simulink model "ADXL345_IMU"  (R2017a)
settings: Solver=FixedStepDiscrete  StartTime=0.0  StopTime=0.01  RelTol=1e-3
PostLoadFcn:
  | ChipSelect = 1;  % choose I2C comms
  | AddressAlt  = 1;  % use default address
  | 
  | if AddressAlt == 1
  | SlvAddr = uint8(hex2dec('1D'));  % ADDR ALT = 1
  | else
  | SlvAddr = uint8(hex2dec('53'));  % ADDR ALT = 0
  | end
  | 
  | AccelXRegAddr = uint8(hex2dec('32'));
  | AccelYRegAddr = uint8(hex2dec('34'));
  | AccelZRegAddr = uint8(hex2dec('36'));
  | 
  | fifoCfgRegAddr = uint8(hex2dec('38'));
  | fifoCfgRegData = uint8(bin2dec('00000100'));
  | 
  | fifoStatusReg = uint8(hex2dec('39'));
  | 
  | deviceAddr = fi(SlvAddr,0,7,0);
settings Model: DataTypeOverride=Off  Creator=skuznick  LastModifiedBy=skuznick
settings DataIOCC: SaveOutput=off  SaveTime=off
settings OptimizationCC: BlockReduction=off  ConditionallyExecuteInputs=off  DefaultParameterBehavior=Inlined
settings DebuggingCC: AlgebraicLoopMsg=error  SingleTaskRateTransMsg=error
settings HardwareCC: ProdBitPerPointer=32  ProdBitPerSizeT=32  ProdBitPerPtrDiffT=32  ProdLargestAtomicFloat=None  ProdIntDivRoundTo=Undefined  ProdEndianess=Unspecified  ProdWordSize=32  ProdHWDeviceType=ASIC/FPGA->ASIC/FPGA  ProdEqTarget=off

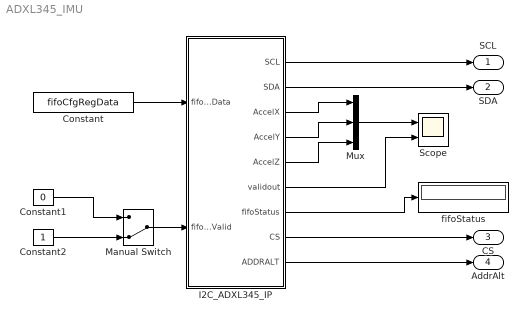
== system ADXL345_IMU ==
  Constant : Constant  Value=fifoCfgRegData  OutDataTypeStr=uint8  SampleTime=1/400e3
  Constant1 : Constant  Value=0  OutDataTypeStr=boolean  SampleTime=-1
  Constant2 : Constant  OutDataTypeStr=boolean  SampleTime=-1
  I2C_ADXL345_IP : Subsystem  TreatAsAtomicUnit=on
  Manual Switch : ManualSwitch  CurrentSetting=0
  Mux : Mux  Inputs=3
  Scope : Scope  NumInputPorts=2
  fifoStatus : Display
  SCL : Outport
  SDA : Outport  Port=2
  CS : Outport  Port=3
  AddrAlt : Outport  Port=4
  wires:
  I2C_ADXL345_IP/2(SDA) -> SDA/1
  I2C_ADXL345_IP/1(SCL) -> SCL/1
  I2C_ADXL345_IP/8(CS) -> CS/1
  I2C_ADXL345_IP/9(ADDRALT) -> AddrAlt/1
  Manual Switch/1 -> I2C_ADXL345_IP/2(fifoCfgValid)
  Constant1/1 -> Manual Switch/1
  Constant2/1 -> Manual Switch/2
  Constant/1 -> I2C_ADXL345_IP/1(fifoCfgData)
  I2C_ADXL345_IP/6(validout) -> Scope/2
  Mux/1 -> Scope/1
  I2C_ADXL345_IP/4(AccelY) -> Mux/2
  I2C_ADXL345_IP/3(AccelX) -> Mux/1
  I2C_ADXL345_IP/5(AccelZ) -> Mux/3
  I2C_ADXL345_IP/7(fifoStatus) -> fifoStatus/1

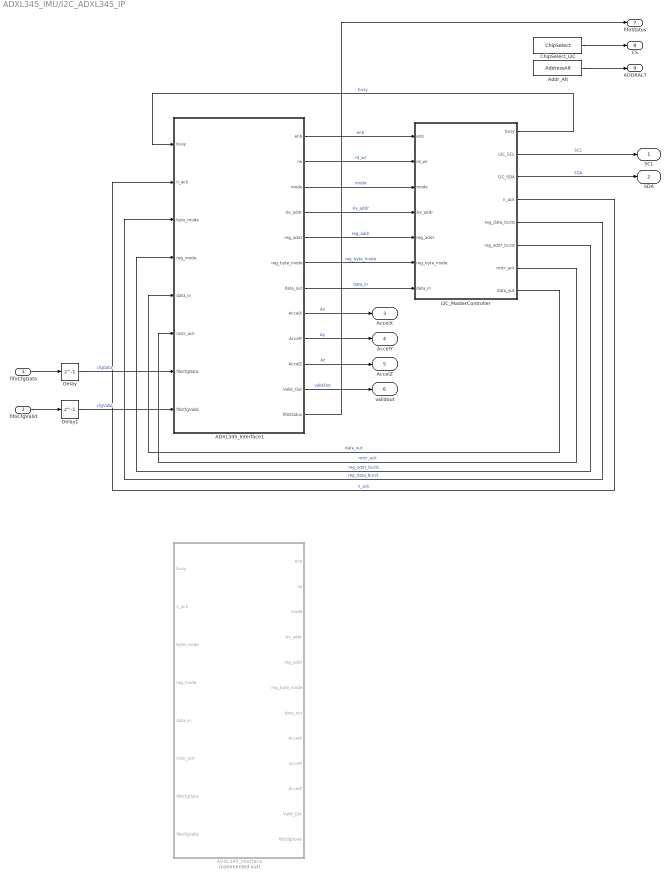
== system ADXL345_IMU/I2C_ADXL345_IP ==
  fifoCfgData : Inport
  fifoCfgValid : Inport  Port=2
  ADXL345_Interface : Stateflow chart  Commented=on  TreatAsAtomicUnit=on
  ADXL345_Interface1 : Stateflow chart  TreatAsAtomicUnit=on
  Addr_Alt : Constant  Value=AddressAlt  OutDataTypeStr=boolean  SampleTime=-1
  ChipSelect_I2C : Constant  Value=ChipSelect  OutDataTypeStr=boolean  SampleTime=-1
  Delay : Delay  DelayLength=1  InitialCondition=0
  Delay1 : Delay  DelayLength=1  InitialCondition=0
  I2C_MasterController : Subsystem
  SCL : Outport
  SDA : Outport  Port=2
  AccelX : Outport  Port=3
  AccelY : Outport  Port=4
  AccelZ : Outport  Port=5
  validout : Outport  Port=6
  fifoStatus : Outport  Port=7
  CS : Outport  Port=8
  ADDRALT : Outport  Port=9
  wires:
  ADXL345_Interface1/7(data_out) -> I2C_MasterController/7(data_in)  "data_in"
  I2C_MasterController/8(data_out) -> ADXL345_Interface1/5(data_in)  "data_out"
  I2C_MasterController/7(mstr_ack) -> ADXL345_Interface1/6(mstr_ack)  "mstr_ack"
  I2C_MasterController/4(n_ack) -> ADXL345_Interface1/2(n_ack)  "n_ack"
  I2C_MasterController/5(reg_data_burst) -> ADXL345_Interface1/3(byte_mode)  "reg_data_burst"
  I2C_MasterController/6(reg_addr_burst) -> ADXL345_Interface1/4(reg_mode)  "reg_addr_burst"
  I2C_MasterController/1(busy) -> ADXL345_Interface1/1(busy)  "busy"
  I2C_MasterController/3(I2C_SDA) -> SDA/1  "SDA"
  I2C_MasterController/2(I2C_SCL) -> SCL/1  "SCL"
  ADXL345_Interface1/6(reg_byte_mode) -> I2C_MasterController/6(reg_byte_mode)  "reg_byte_mode"
  ADXL345_Interface1/5(reg_addr) -> I2C_MasterController/5(reg_addr)  "reg_addr"
  ADXL345_Interface1/4(slv_addr) -> I2C_MasterController/4(slv_addr)  "slv_addr"
  ADXL345_Interface1/3(mode) -> I2C_MasterController/3(mode)  "mode"
  ADXL345_Interface1/2(rw) -> I2C_MasterController/2(rd_wr)  "rd_wr"
  ADXL345_Interface1/1(enb) -> I2C_MasterController/1(enb)  "enb"
  Delay/1 -> ADXL345_Interface1/7(fifoCfgData)  "cfgData"
  Delay1/1 -> ADXL345_Interface1/8(fifoCfgValid)  "cfgValid"
  fifoCfgData/1 -> Delay/1
  fifoCfgValid/1 -> Delay1/1
  ChipSelect_I2C/1 -> CS/1
  Addr_Alt/1 -> ADDRALT/1
  ADXL345_Interface1/9(AccelY) -> AccelY/1  "Ay"
  ADXL345_Interface1/10(AccelZ) -> AccelZ/1  "Az"
  ADXL345_Interface1/11(Valid_Out) -> validout/1  "validOut"
  ADXL345_Interface1/8(AccelX) -> AccelX/1  "Ax"
  ADXL345_Interface1/12(fifoStatus) -> fifoStatus/1

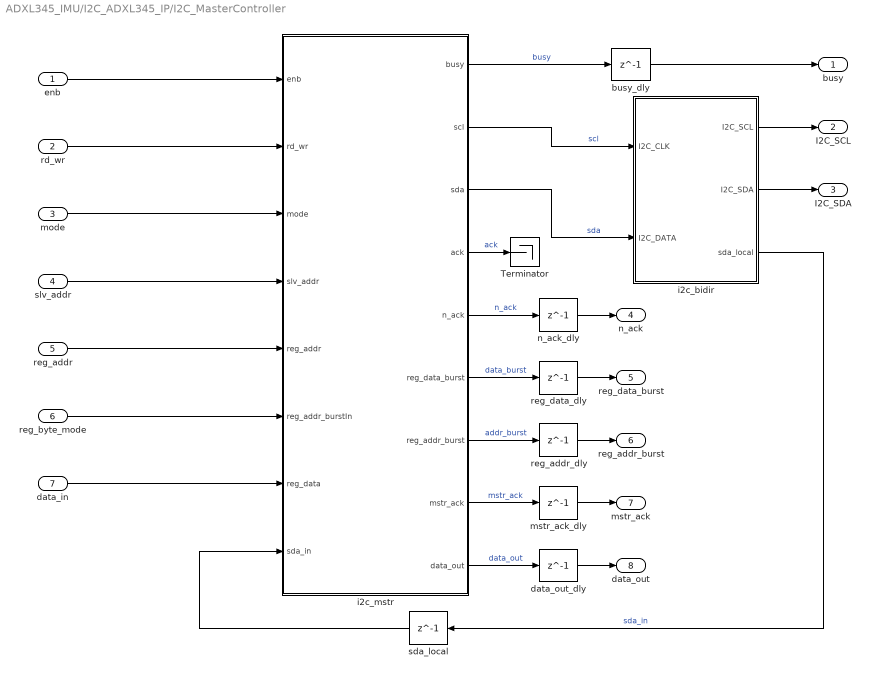
== system ADXL345_IMU/I2C_ADXL345_IP/I2C_MasterController ==
  enb : Inport
  rd_wr : Inport  Port=2
  mode : Inport  Port=3
  slv_addr : Inport  Port=4
  reg_addr : Inport  Port=5
  reg_byte_mode : Inport  Port=6
  data_in : Inport  Port=7
  Terminator : Terminator
  busy_dly : Delay  DelayLength=1
  data_out_dly : Delay  DelayLength=1
  i2c_bidir : Subsystem  TreatAsAtomicUnit=on
  i2c_mstr : Stateflow chart  TreatAsAtomicUnit=on
  mstr_ack_dly : Delay  DelayLength=1
  n_ack_dly : Delay  DelayLength=1
  reg_addr_dly : Delay  DelayLength=1
  reg_data_dly : Delay  DelayLength=1
  sda_local : Delay  DelayLength=1
  busy : Outport
  I2C_SCL : Outport  Port=2
  I2C_SDA : Outport  Port=3
  n_ack : Outport  Port=4
  reg_data_burst : Outport  Port=5
  reg_addr_burst : Outport  Port=6
  mstr_ack : Outport  Port=7
  data_out : Outport  Port=8
  wires:
  data_out_dly/1 -> data_out/1
  mstr_ack_dly/1 -> mstr_ack/1
  i2c_mstr/9(data_out) -> data_out_dly/1  "data_out"
  i2c_mstr/8(mstr_ack) -> mstr_ack_dly/1  "mstr_ack"
  busy_dly/1 -> busy/1
  n_ack_dly/1 -> n_ack/1
  reg_data_dly/1 -> reg_data_burst/1
  reg_addr_dly/1 -> reg_addr_burst/1
  i2c_mstr/1(busy) -> busy_dly/1  "busy"
  rd_wr/1 -> i2c_mstr/2(rd_wr)
  mode/1 -> i2c_mstr/3(mode)
  data_in/1 -> i2c_mstr/7(reg_data)
  enb/1 -> i2c_mstr/1(enb)
  slv_addr/1 -> i2c_mstr/4(slv_addr)
  reg_byte_mode/1 -> i2c_mstr/6(reg_addr_burstIn)
  reg_addr/1 -> i2c_mstr/5(reg_addr)
  i2c_bidir/1(I2C_SCL) -> I2C_SCL/1
  i2c_bidir/2(I2C_SDA) -> I2C_SDA/1
  i2c_mstr/4(ack) -> Terminator/1  "ack"
  i2c_mstr/2(scl) -> i2c_bidir/1(I2C_CLK)  "scl"
  i2c_bidir/3(sda_local) -> sda_local/1  "sda_in"
  sda_local/1 -> i2c_mstr/8(sda_in)
  i2c_mstr/3(sda) -> i2c_bidir/2(I2C_DATA)  "sda"
  i2c_mstr/5(n_ack) -> n_ack_dly/1  "n_ack"
  i2c_mstr/6(reg_data_burst) -> reg_data_dly/1  "data_burst"
  i2c_mstr/7(reg_addr_burst) -> reg_addr_dly/1  "addr_burst"

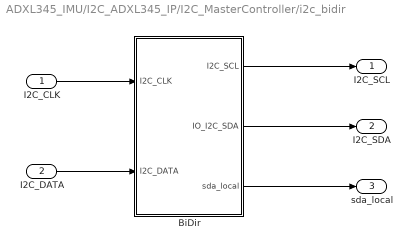
== system ADXL345_IMU/I2C_ADXL345_IP/I2C_MasterController/i2c_bidir ==
  I2C_CLK : Inport
  I2C_DATA : Inport  Port=2
  BiDir : Subsystem  TreatAsAtomicUnit=on
  I2C_SCL : Outport
  I2C_SDA : Outport  Port=2
  sda_local : Outport  Port=3
  wires:
  BiDir/2(IO_I2C_SDA) -> I2C_SDA/1
  I2C_CLK/1 -> BiDir/1(I2C_CLK)
  I2C_DATA/1 -> BiDir/2(I2C_DATA)
  BiDir/1("I2C_SCL ") -> I2C_SCL/1
  BiDir/3(sda_local) -> sda_local/1

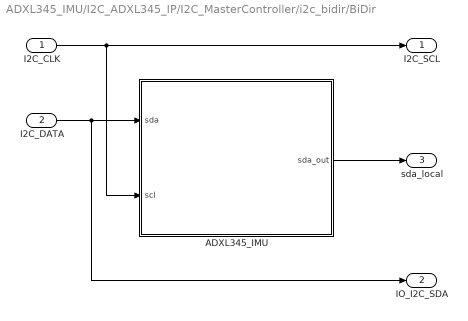
== system ADXL345_IMU/I2C_ADXL345_IP/I2C_MasterController/i2c_bidir/BiDir ==
  I2C_CLK : Inport  OutDataTypeStr=boolean
  I2C_DATA : Inport  Port=2  OutDataTypeStr=boolean
  ADXL345_IMU : Stateflow chart  TreatAsAtomicUnit=on
  "I2C_SCL " : Outport  OutDataTypeStr=boolean
  IO_I2C_SDA : Outport  Port=2  OutDataTypeStr=boolean
  sda_local : Outport  Port=3  OutDataTypeStr=boolean
  wires:
  ADXL345_IMU/1(sda_out) -> sda_local/1
  I2C_CLK/1 -> "I2C_SCL "/1, ADXL345_IMU/2(scl)
  I2C_DATA/1 -> IO_I2C_SDA/1, ADXL345_IMU/1(sda)

== stateflow chart ADXL345_IMU/I2C_ADXL345_IP/ADXL345_Interface1 ==
  settings: executeAtInitialization=1
  state init
    %initstate
    Valid_Out = false;
  note: I2C Configuration for ADXL345
  state idle
    %idlestate
    enb 	= 0;
    rw 		= 0;
    mode 	= 0;
    inc_in  = 0;
    wait 	= 0;
    cnt = 0;
    reg_byte_mode = 0;
  note: 0x32 50 DATAX0 R 00000000 X-Axis Data 0
      | 0x33 51 DATAX1 R 00000000 X-Axis Data 1
      | 0x34 52 DATAY0 R 00000000 Y-Axis Data 0
      | 0x35 53 DATAY1 R 00000000 Y-Axis Data 1
      | 0x36 54 DATAZ0 R 00000000 Z-Axis Data 0
      | 0x37 55 DATAZ1 R 00000000 Z-Axis Data 1
  state set_config [commented out]
    enb = 1;
    rw = 0;
    mode = 0;
    reg_byte_mode = 0;
    slv_addr = SlvAddr;
    reg_addr = fifoCfgRegAddr;
    data_out = fifoCfgData;
  state waitforNotBusy [commented out]
  state getFifoStatus [commented out]
    entry:
    enb = 1;
    rw = 1;
    mode = 0;
    slv_addr = SlvAddr;
    reg_addr =  fifoStatusReg;
  state read_fifoReg [commented out]
    fifoStatus = uint8(data_in);
  note: fifoStatus is an example of
      | doing a 1-byte READ
  state check_cfg
    en: enb = 0;
  state read_accelX_registers0
    entry:
    enb = 1;
    rw = 1;
    mode = 1;
    slv_addr = SlvAddr;
    reg_byte_mode = 0;
    reg_addr =  AccelXRegAddr;
    Valid_Out = false;
  state accelX_LSB
    enb = 1;
    tempVal = uint16(data_in);
  state toggle
    mode = 0;
  state accelX_MSB
    enb = 0;
    AccelX = tempVal + uint16(data_in << 8);
  state read_accelY_registers0
    enb = 1;
    rw = 1;
    mode = 1;
    slv_addr = SlvAddr;
    reg_byte_mode = 0;
    reg_addr =  AccelYRegAddr;
  state accelY_LSB
    enb = 1;
    tempVal = uint16(data_in);
  state toggle1
    mode = 0;
  state accelY_MSB
    enb = 0;
    AccelY = tempVal + uint16(data_in << 8);
  state read_accelZ_registers0
    enb = 1;
    rw = 1;
    mode = 1;
    slv_addr = SlvAddr;
    reg_byte_mode = 0;
    reg_addr =  AccelZRegAddr;
  state accelZ_LSB
    enb = 1;
    tempVal = uint16(data_in);
  state toggle2
    mode = 0;
  state accelZ_MSB
    enb = 0;
    AccelZ = tempVal + uint16(data_in << 8);
  state Valid
    en: enb = 0;
    cnt = 0;
    Valid_Out = 1;
    du: cnt = cnt + 1;
  (default) -> init
  init -> idle
  check_cfg -> idle
  accelX_LSB -> idle [order 1] : [n_ack==1]
  idle -> set_config [commented out] : [busy==0 & fifoCfgValid == 1]
  idle -> read_accelX_registers0
  set_config -> waitforNotBusy [commented out] : [busy==1]
  waitforNotBusy -> getFifoStatus [commented out] : [busy==0]
  getFifoStatus -> read_fifoReg [commented out] : [mstr_ack==1]
  read_fifoReg -> read_accelX_registers0 [commented out] : [busy==0]
  read_accelX_registers0 -> check_cfg [order 2] : [n_ack == 1]
  accelX_MSB -> check_cfg [order 2] : [n_ack==1]
  accelZ_MSB -> check_cfg [order 1] : [n_ack==1]
  Valid -> check_cfg : [cnt >= 1000]
  accelY_MSB -> check_cfg [order 2] : [n_ack==1]
  read_accelX_registers0 -> accelX_LSB [order 1] : [mstr_ack==1]
  accelX_LSB -> toggle [order 2] : [mstr_ack==0]
  toggle -> accelX_MSB : [mstr_ack==1]
  accelX_MSB -> read_accelY_registers0 [order 1] : [busy==0]
  read_accelY_registers0 -> accelY_LSB : [mstr_ack==1]
  accelY_LSB -> toggle1 : [mstr_ack==0]
  toggle1 -> accelY_MSB : [mstr_ack==1]
  accelY_MSB -> read_accelZ_registers0 [order 1] : [busy==0 & n_ack==0]
  read_accelZ_registers0 -> accelZ_LSB : [mstr_ack==1]
  accelZ_LSB -> toggle2 : [mstr_ack==0]
  toggle2 -> accelZ_MSB : [mstr_ack==1]
  accelZ_MSB -> Valid [order 2]
  data: enb output boolean size=1; rw output boolean size=1; mode output boolean size=1; slv_addr output uint8; reg_addr output uint8; reg_byte_mode output boolean size=1; data_out output uint8; busy input; inc_in local uint8; n_ack input; byte_mode input boolean size=1; reg_mode input boolean size=1; cnt local uint32; wait local uint16; data_in input uint8 size=1; mstr_ack input; AccelX output uint16; AccelY output uint16; AccelZ output uint16; SlvAddr parameter uint8; AccelXRegAddr parameter uint8; AccelYRegAddr parameter uint8; AccelZRegAddr parameter uint8; Valid_Out output boolean; fifoCfgRegAddr parameter uint8; fifoCfgData input uint8; fifoCfgValid input boolean; tempVal local uint16; fifoStatus output uint8; fifoStatusReg parameter uint8

== stateflow chart ADXL345_IMU/I2C_ADXL345_IP/I2C_MasterController/i2c_mstr ==
  settings: executeAtInitialization=1
  note: I2C Master Controller
  state idle
    entry:
    scl(:) = 1;
    sda(:) = 1;
    busy(:)  = 0;
  state stop_ext
    entry:
    scl (:) = 1;
    sda(:) = 1;
    ack(:) = 0;
  state ready
    entry:
    scl(:) = 1;
    sda(:) = 1;
    data_out(:) = 0;
  state stop
    entry:
    sda(:) = 0;
  state start_n
    entry:
    scl(:) = 1;
    sda(:) = 0;
    bit_cnt(:) = 7;
    busy(:) = 1;
    reg_byte_cnt =1;
  state scl_ext_p
    entry:
    scl(:) = 1;
    sda(:) = 0;
    ack(:) = 0;
  state start_p
    entry:
    sda(:) = 0;
  state scl_ext_n
    entry:
    scl(:) = 0;
    sda(:) = 0;
    ack(:) = 0;
    mstr_ack(:) = 0;
  state Increment_Byte_count1
    entry:
    scl(:) = 1;
    bit_cnt = 8;
    mstr_ack(:) =0;
    reg_data_burst(:) = 1;
    data_out(:) = 0;
  state mastr_ack_data_cnf
    entry:
    scl(:) = 1;
    sda(:) = 0;
    mstr_ack (:) = 1;
  state cmd_slave_addr_n
    entry:
    scl(:) = 0;
    sda(:) = bitget(slv_addr(:),bit_cnt);
  state ack_data_cnf
    entry:
    scl(:) = 1;
    ack (:) = 1;
  state cmd_slave_addr_p
    entry:
    scl(:) = 1;
    bit_cnt = bit_cnt-1;
  state Increment_Byte_count
    entry:
    scl(:) = 1;
    bit_cnt = 8;
    ack (:) = 1;
    reg_data_burst(:) = 1;
  state mastr_ack_data
    entry:
    scl(:) = 0;
    sda(:) = 0;
    mstr_ack(:) = 1;
  state write_n
    entry:
    scl(:) = 0;
    sda(:) = 0;
  state ack_data
    entry:
    scl(:) = 0;
    sda(:) = 1;
    ack(:) = 1;
  state cmd_reg_read_data_p
    entry:
    scl(:) = 1;
    bit_cnt = bit_cnt-1;
  state write_p
    entry:
    scl(:) = 1;
    sda(:) = 0;
  state cmd_reg_data_p
    entry:
    scl(:) = 1;
    bit_cnt = bit_cnt-1;
  state ack_slv
    entry:
    scl(:) = 0;
    ack(:) = 1;
    sda(:) = 1;
  state error_ack
    entry:
    scl(:) = 0;
    sda(:) = 1;
    n_ack(:) = 1;
  state cmd_reg_read_data_n
    entry:
    scl(:) = 0;
    if sda_in == 1;
    data_out = bitset(data_out,bit_cnt);
    end
    %data_out(bit_cnt) = sda_in;
    %mstr_ack(:) = 0
    ack(:) = 0;
  state ack_slv_cnf
    entry:
    scl(:)= 1;
    ack(:) = 1;
    bit_cnt = 8;
  state cmd_reg_data_n
    entry:
    scl(:) = 0;
    sda(:) = bitget(reg_data,bit_cnt);
    ack(:) = 0;
    reg_data_burst(:) = 0;
  state ack_addr_m_cnf
    entry:
    scl(:) = 1;
    bit_cnt = 8;
    ack(:) = 1;
  state cmd_reg_addr_n
    entry:
    scl(:) = 0;
    ack(:) = 0;
    sda(:) = bitget(reg_addr,bit_cnt);
    reg_addr_burst(:)=0;
  state delay
    entry:
    scl(:) = 0;
    sda(:) = 1;
  state repeat_strt_n
    entry:
    scl(:) = 1;
    sda(:) = 0;
    bit_cnt(:) = 7;
    busy(:) = 1;
    reg_byte_cnt =1;
  state cmd_reg_addr_p
    entry:
    scl(:)= 1;
    bit_cnt = bit_cnt-1;
  state ready_repeated
    entry:
    scl(:) = 1;
    sda(:) = 1;
  state ack_addr_m
    entry:
    scl(:) = 0;
    ack (:) = 1;
    sda(:) = 1;
  state repeat_strt_p
    entry:
    sda(:) = 0;
  state ready_repeated_dummy
    entry:
    scl(:) = 1;
    sda(:) = 1;
  state ack_addrm1
    entry:
    scl(:) = 1;
    ack(:) = 1;
    bit_cnt = 8;
    reg_addr_burst(:)=1;
  state cmd_slave_addr_n1
    entry:
    scl(:) = 0;
    sda(:) = bitget(slv_addr(:),bit_cnt);
  state cmd_slave_addr_p1
    entry:
    scl(:) = 1;
    bit_cnt = bit_cnt-1;
  state read_n
    entry:
    scl(:) = 0;
    sda(:) = 1;
  state read_p
    entry:
    scl(:) = 1;
    sda(:) = 1;
    bit_cnt = 8;
  state ack_slv1
    entry:
    scl(:) = 0;
    ack(:) = 1;
    sda(:) = 1;
  state ack_slv_cnf1
    entry:
    scl(:)= 1;
    ack(:) = 1;
    bit_cnt = 8;
  (default) -> idle
  stop_ext -> idle
  error_ack -> idle
  idle -> ready : [enb==1]
  stop -> stop_ext
  ready -> start_n
  scl_ext_p -> stop
  start_n -> start_p
  scl_ext_n -> scl_ext_p
  start_p -> cmd_slave_addr_n
  mastr_ack_data_cnf -> scl_ext_n [order 2]
  mastr_ack_data_cnf -> Increment_Byte_count1 [order 1] : [mode ==1]
  cmd_slave_addr_p -> cmd_slave_addr_n [order 1] : [bit_cnt > 0]
  ack_data_cnf -> scl_ext_n
  cmd_slave_addr_n -> cmd_slave_addr_p
  mastr_ack_data -> mastr_ack_data_cnf
  Increment_Byte_count1 -> cmd_reg_read_data_n
  ack_data -> ack_data_cnf [order 2] : [sda_in == 0]
  cmd_slave_addr_p -> write_n [order 2]
  Increment_Byte_count -> cmd_reg_data_n
  cmd_reg_read_data_p -> mastr_ack_data [order 2]
  ack_data -> Increment_Byte_count [order 1] : [mode == 1]
  ack_data -> error_ack [order 3]
  write_n -> write_p
  cmd_reg_read_data_p -> cmd_reg_read_data_n [order 1] : [bit_cnt > 0]
  cmd_reg_data_p -> ack_data [order 2]
  cmd_reg_read_data_n -> cmd_reg_read_data_p
  write_p -> ack_slv
  ack_slv -> error_ack [order 2]
  cmd_reg_data_p -> cmd_reg_data_n [order 1] : [bit_cnt > 0]
  cmd_reg_data_n -> cmd_reg_data_p
  ack_slv -> ack_slv_cnf [order 1] : [sda_in == 0]
  ack_addr_m -> error_ack [order 3]
  ack_slv1 -> error_ack [order 2]
  ack_slv_cnf1 -> cmd_reg_read_data_n
  ack_slv_cnf -> cmd_reg_addr_n
  ack_addr_m -> ack_addr_m_cnf [order 2] : [sda_in == 0]
  ack_addr_m_cnf -> cmd_reg_data_n [order 1] : [rd_wr ==0]
  ack_addrm1 -> cmd_reg_addr_n
  ack_addr_m_cnf -> delay [order 2] : [rd_wr == 1]
  cmd_reg_addr_p -> cmd_reg_addr_n [order 1] : [bit_cnt > 0]
  cmd_reg_addr_n -> cmd_reg_addr_p
  delay -> ready_repeated
  ready_repeated_dummy -> repeat_strt_n
  cmd_reg_addr_p -> ack_addr_m [order 2]
  repeat_strt_n -> repeat_strt_p
  ready_repeated -> ready_repeated_dummy
  ack_addr_m -> ack_addrm1 [order 1] : [reg_addr_burstIn ==1]
  repeat_strt_p -> cmd_slave_addr_n1
  cmd_slave_addr_p1 -> cmd_slave_addr_n1 [order 1] : [bit_cnt > 0]
  cmd_slave_addr_n1 -> cmd_slave_addr_p1
  cmd_slave_addr_p1 -> read_n [order 2]
  read_n -> read_p
  read_p -> ack_slv1
  ack_slv1 -> ack_slv_cnf1 [order 1] : [sda_in == 0]
  data: enb input boolean size=1; rd_wr input boolean size=1; mode input boolean size=1; busy output boolean size=1; bit_cnt local uint8; scl output boolean size=1; sda output boolean size=1; slv_addr input uint8; reg_addr input uint8; reg_addr_burstIn input boolean size=1; reg_data input uint8; sda_in input boolean size=1; ack output boolean size=1; n_ack output boolean size=1; reg_byte_cnt local uint8; reg_data_burst output boolean size=1; reg_addr_burst output boolean size=1; mstr_ack output boolean size=1; data_out output fixdt(0,8,0) size=1

== stateflow chart ADXL345_IMU/I2C_ADXL345_IP/ADXL345_Interface ==
  settings: executeAtInitialization=1
  state init
    %initstate
    enb 	= 0;
    rw 		= 0;
    mode 	= 0;
    inc_in  = 0;
    wait 	= 0;
    cnt = 0;
    Valid_Out = false;
    fifoCfgDone = 0;
  state set_config
    enb = 1;
    rw = 0;
    mode = 0;
    reg_byte_mode = 0;
    slv_addr = SlvAddr;
    reg_addr = fifoCfgRegAddr;
    data_out = fifoCfgData;
  note: I2C Configuration for ADXL345
  note: 0x32 50 DATAX0 R 00000000 X-Axis Data 0
      | 0x33 51 DATAX1 R 00000000 X-Axis Data 1
      | 0x34 52 DATAY0 R 00000000 Y-Axis Data 0
      | 0x35 53 DATAY1 R 00000000 Y-Axis Data 1
      | 0x36 54 DATAZ0 R 00000000 Z-Axis Data 0
      | 0x37 55 DATAZ1 R 00000000 Z-Axis Data 1
  state read_accelX_registers
    fifoCfgDone = 1;
    enb = 1;
    rw = 1;
    mode = 1;
    slv_addr = SlvAddr;
    reg_byte_mode = 0;
    reg_addr =  AccelXRegAddr;
  state check_cfg
    en: enb = 0;
    fifoCfgDone = 0;
  state accelX_HSB
    enb = 0;
    AccelX = AccelX & (data_in << 8);
  state accelX_LSB
    enb=1;
    mode = 0;
    AccelX = uint16(data_in);
  state read_accelY_registers
    enb = 1;
    rw = 1;
    mode = 1;
    slv_addr = SlvAddr;
    reg_byte_mode = 0;
    reg_addr =  AccelYRegAddr;
  state accelY_LSB
    enb = 1;
    mode = 0;
    AccelY = data_in;
  state accelY_HSB
    enb = 0;
    AccelY = AccelY & (data_in << 8);
  state read_accelZ_registers
    enb = 1;
    rw = 1;
    mode = 1;
    slv_addr = SlvAddr;
    reg_byte_mode = 0;
    reg_addr =  AccelZRegAddr;
  state accelZ_LSB
    enb = 1;
    mode = 0;
    AccelZ = uint16(data_in);
  state accelZ_HSB
    enb = 0;
    AccelZ = AccelZ & (data_in << 8);
  state Valid
    en: enb = 0;
    cnt = 0;
    Valid_Out = 1;
    du: cnt = cnt + 1;
  (default) -> init
  init -> set_config : [busy==0]
  read_accelX_registers -> init [order 2] : [n_ack == 1]
  set_config -> init [order 2] : [n_ack == 1]
  set_config -> read_accelX_registers [order 1] : [busy==0 & n_ack == 0]
  check_cfg -> set_config [order 1] : [fifoCfgValid == 1]
  check_cfg -> read_accelX_registers [order 2]
  read_accelX_registers -> accelX_LSB [order 1] : [mstr_ack==1 ]
  accelX_LSB -> read_accelX_registers [order 2] : [n_ack==1]
  Valid -> check_cfg : [cnt >= 500]
  accelX_HSB -> read_accelX_registers [order 1] : [n_ack == 1]
  accelX_LSB -> accelX_HSB [order 1] : [byte_mode == 1& mstr_ack==1]
  accelX_HSB -> read_accelY_registers [order 2] : [busy==0 & n_ack == 0]
  read_accelY_registers -> accelY_LSB : [mstr_ack==1 ]
  accelY_LSB -> read_accelY_registers [order 2] : [n_ack==1]
  accelY_HSB -> read_accelY_registers [order 1] : [n_ack == 1]
  accelY_LSB -> accelY_HSB [order 1] : [byte_mode == 1& mstr_ack==1]
  accelY_HSB -> read_accelZ_registers [order 2] : [busy==0 & n_ack == 0]
  read_accelZ_registers -> accelZ_LSB : [mstr_ack == 1 ]
  accelZ_LSB -> read_accelZ_registers [order 1] : [n_ack==1]
  accelZ_HSB -> read_accelZ_registers [order 1] : [n_ack == 1]
  accelZ_LSB -> accelZ_HSB [order 2] : [byte_mode == 1& mstr_ack==1]
  accelZ_HSB -> Valid [order 2] : [busy==0 & n_ack == 0]
  data: enb output boolean size=1; rw output boolean size=1; mode output boolean size=1; slv_addr output uint8; reg_addr output uint8; reg_byte_mode output boolean size=1; data_out output uint8; busy input; inc_in local uint8; n_ack input; byte_mode input boolean size=1; reg_mode input boolean size=1; cnt local uint32; wait local uint16; data_in input uint8 size=1; mstr_ack input; AccelX output uint16; AccelY output uint16; AccelZ output uint16; SlvAddr parameter uint8; AccelXRegAddr parameter uint8; AccelYRegAddr parameter uint8; AccelZRegAddr parameter uint8; Valid_Out output boolean; fifoCfgRegAddr parameter uint8; fifoCfgRegData parameter uint8; fifoCfgData input uint8; fifoCfgValid input boolean; fifoCfgDone output boolean

== stateflow chart ADXL345_IMU/I2C_ADXL345_IP/I2C_MasterController/i2c_bidir/BiDir/ADXL345_IMU ==
  state init
    entry:
    rd_cnt = 0;
    reg_idx = 0;
  state regdata = sendregdata(reg) [function]
    (default) -> (junction 86)
    (junction 86) -> (junction 89) [order 1] : [reg ==AccelXRegAddr]
    (junction 86) -> (junction 88) [order 2]
    (junction 89) -> (junction 90) : {regdata = hex2dec('D2');}
    (junction 90) -> (junction 99)
    (junction 99) -> (junction 112)
    (junction 88) -> (junction 97) [order 1] : [reg==AccelYRegAddr]
    (junction 97) -> (junction 111) : {regdata = hex2dec('E1');}
    (junction 88) -> (junction 91) [order 2]
    (junction 111) -> (junction 112)
    (junction 112) -> (junction 103)
    (junction 91) -> (junction 106) [order 1] : [reg==AccelZRegAddr]
    (junction 106) -> (junction 109) : {regdata=hex2dec('2E');}
    (junction 91) -> (junction 127) [order 2]
    (junction 109) -> (junction 103)
    (junction 103) -> (junction 143)
    (junction 127) -> (junction 126) [order 1] : [reg ==AccelXRegAddr+1]
    (junction 127) -> (junction 128) [order 2]
    (junction 126) -> (junction 131) : {regdata = hex2dec('04');}
    (junction 131) -> (junction 143)
    (junction 143) -> (junction 130)
    (junction 128) -> (junction 142) [order 1] : [reg==AccelYRegAddr+1]
    (junction 142) -> (junction 154) : {regdata = hex2dec('10');}
    (junction 128) -> (junction 140) [order 2]
    (junction 154) -> (junction 130)
    (junction 130) -> (junction 149)
    (junction 140) -> (junction 141) [order 1] : [reg==AccelZRegAddr+1]
    (junction 141) -> (junction 153) : {regdata=hex2dec('16');}
    (junction 140) -> (junction 196) [order 2]
    (junction 153) -> (junction 149)
    (junction 149) -> (junction 197)
    (junction 196) -> (junction 194) [order 1] : [reg==fifoStatusReg]
    (junction 194) -> (junction 192) : {regdata=hex2dec('FE');}
    (junction 196) -> (junction 152) [order 2] : {regdata=0;}
    (junction 192) -> (junction 197)
    (junction 197) -> (junction 152)
  state idle
    entry:
    sda_out = false;
    addr = fi(0,0,7,0);
    data = fi(0,0,8,0);
  state start
    en:
    bit_idx(:) = 7;
  state startgetaddr
  state getaddr
    entry:
    if sda == 1
    addr = bitset(addr,bit_idx);
    end
    bit_idx = bit_idx - 1;
  note: RegX (0x32/0x33) = 1234 (0x04d2)
      | RegY (0x34/0x35) = 4321 (0x10e1)
      | RegZ (0x36/0x37) = 5678 (0x162e)
  state endgetaddr
    entry: rw = sda;
  state sendack
    entry:
    sda_out(:) = 0;
    bit_idx = 8;
  state senddatastart
    entry: data(:) = sendregdata(reg_idx+rd_cnt);
    bit_idx = 8;
    sda_out(:) = bitget(data,bit_idx);
    bit_idx = bit_idx - 1;
  state waitForNack
  state getdatastart
  state sendbyte
    entry: sda_out(:) = bitget(data,bit_idx);
  state getdata
    entry:
    if sda == 1
    data = bitset(data,bit_idx);
    end
    bit_idx = bit_idx - 1;
  state sendbit
    entry: bit_idx = bit_idx - 1;
  state endgetdata
    entry:
    reg_idx = uint8(data);
  state waitstop
  state getcfgregstart
  state getcfgdata
    entry:
    if sda == 1
    data = bitset(data,bit_idx);
    end
    bit_idx = bit_idx - 1;
  state endgetcfgdata
    entry:
    %data
    sda_out(:) = 0;
    % setregister(data)
  (default) -> init
  init -> idle
  endgetaddr -> idle [order 1] : [addr ~= deviceAddr]
  waitForNack -> idle : [scl==1 & sda==1]
  endgetdata -> idle [order 1] : [reg_idx ~= fifoCfgRegAddr]
  idle -> start : [scl == 1 & sda == 0]
  start -> startgetaddr : [scl == 1]
  getaddr -> startgetaddr [order 1] : [bit_idx > 0]
  startgetaddr -> getaddr : [scl==1]
  getaddr -> endgetaddr [order 2] : [scl==1]
  endgetaddr -> sendack [order 2]
  sendack -> senddatastart [order 1] : [scl==1 & rw==1]
  sendack -> getdatastart [order 2] : [scl == 1] {rd_cnt=0;}
  waitstop -> senddatastart [order 2] : [scl==1] {rd_cnt = rd_cnt + 1;}
  senddatastart -> sendbyte
  endgetcfgdata -> waitForNack
  waitstop -> waitForNack [order 1] : [scl==0 & sda==0]
  getdata -> getdatastart [order 1] : [bit_idx > 0]
  getdatastart -> getdata : [scl == 1]
  sendbit -> sendbyte [order 1] : [bit_idx > 0]
  sendbyte -> sendbit : [scl==1]
  getdata -> endgetdata [order 2]
  sendbit -> waitstop [order 2] : [scl==1 & sda==0]
  endgetdata -> getcfgregstart [order 2] : [scl==1] {bit_idx(:) = 8;
      |                 data(:) = 0;}
  getcfgdata -> getcfgregstart [order 1] : [bit_idx > 0]
  getcfgregstart -> getcfgdata : [scl == 1]
  getcfgdata -> endgetcfgdata [order 2]
  data: reg function_input; regdata function_output; sda input boolean; scl input boolean; sda_out output boolean; addr local fixdt(0,7,0) size=1; bit_idx local uint8; deviceAddr parameter fixdt(0,7,0); data local fixdt(0,8,0) size=1; rw local boolean; reg_idx local uint8; rd_cnt local uint8; fifoCfgRegAddr parameter; fifoStatusReg parameter uint8; AccelXRegAddr parameter uint8; AccelYRegAddr parameter uint8; AccelZRegAddr parameter uint8
